simulink model "F16model"  (R2019b)
settings: Solver=ode45  StartTime=0.0  StopTime=150  RelTol=1e-7
values from neighbouring files (symbols this model uses):
  A = [ 0.005142  23.0402  -48.8785  -32.0915  0 0 0 0 0 ... (first row only)    [Final_projectMCT.m]
  B = [  1.585175  1.585175 -1.049275  -1.049275  0 0 ... (first row only)    [Final_projectMCT.m]
  KF = inv(G)*Bs'*S    [Final_projectMCT.m]
settings Model: Creator=harshireddy  LastModifiedBy=jyoth
settings SFSimCC: CustomCodeUndefinedFunction=UseInterfaceOnly

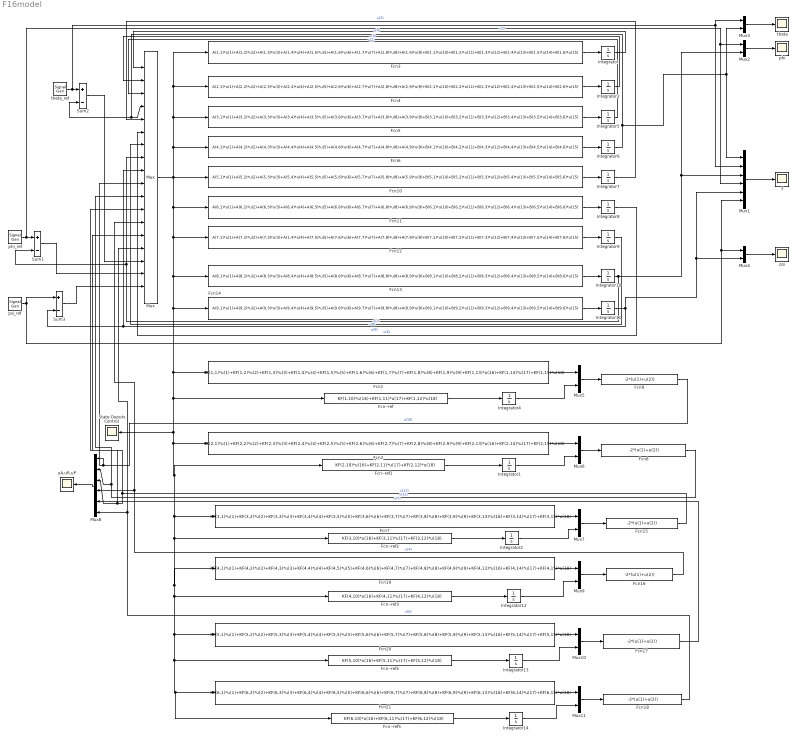
== system F16model ==
  Fcn--ref : Fcn  Expr=KF(1,10)*u(16)+KF(1,11)*u(17)+KF(1,12)*u(18)
  Fcn--ref1 : Fcn  Expr=KF(2,10)*u(16)+KF(2,11)*u(17)+KF(2,12)*u(18)
  Fcn--ref2 : Fcn  Expr=KF(3,10)*u(16)+KF(3,11)*u(17)+KF(3,12)*u(18)
  Fcn--ref3 : Fcn  Expr=KF(4,10)*u(16)+KF(4,11)*u(17)+KF(4,12)*u(18)
  Fcn--ref4 : Fcn  Expr=KF(5,10)*u(16)+KF(5,11)*u(17)+KF(5,12)*u(18)
  Fcn--ref5 : Fcn  Expr=KF(6,10)*u(16)+KF(6,11)*u(17)+KF(6,12)*u(18)
  Fcn1 : Fcn  Expr=KF(1,1)*u(1)+KF(1,2)*u(2)+KF(1,3)*u(3)+KF(1,4)*u(4)+KF(1,5)*u(5)+KF(1,6)*u(6)+KF(1,7)*u(7)+KF(1,8)*u(8)+KF(1,9)*u(9)+KF(1,13)*u(16)+KF(1,14)*u(17)+KF(1,15)*u(18)
  Fcn10 : Fcn  Expr=A(5,1)*u(1)+A(5,2)*u(2)+A(5,3)*u(3)+A(5,4)*u(4)+A(5,5)*u(5)+A(5,6)*u(6)+A(5,7)*u(7)+A(5,8)*u(8)+A(5,9)*u(9)+B(5,1)*u(10)+B(5,2)*u(11)+B(5,3)*u(12)+B(5,4)*u(13)+B(5,5)*u(14)+B(5,6)*u(15)
  Fcn11 : Fcn  Expr=A(6,1)*u(1)+A(6,2)*u(2)+A(6,3)*u(3)+A(6,4)*u(4)+A(6,5)*u(5)+A(6,6)*u(6)+A(6,7)*u(7)+A(6,8)*u(8)+A(6,9)*u(9)+B(6,1)*u(10)+B(6,2)*u(11)+B(6,3)*u(12)+B(6,4)*u(13)+B(6,5)*u(14)+B(6,6)*u(15)
  Fcn12 : Fcn  Expr=A(7,1)*u(1)+A(7,2)*u(2)+A(7,3)*u(3)+A(1,4)*u(4)+A(7,5)*u(5)+A(7,6)*u(6)+A(7,7)*u(7)+A(7,8)*u(8)+A(7,9)*u(9)+B(7,1)*u(10)+B(7,2)*u(11)+B(7,3)*u(12)+B(7,4)*u(13)+B(7,5)*u(14)+B(7,6)*u(15)
  Fcn13 : Fcn  Expr=A(8,1)*u(1)+A(8,2)*u(2)+A(8,3)*u(3)+A(8,4)*u(4)+A(8,5)*u(5)+A(8,6)*u(6)+A(8,7)*u(7)+A(8,8)*u(8)+A(8,9)*u(9)+B(8,1)*u(10)+B(8,2)*u(11)+B(8,3)*u(12)+B(8,4)*u(13)+B(8,5)*u(14)+B(8,6)*u(15)
  Fcn14 : Fcn  Expr=A(9,1)*u(1)+A(9,2)*u(2)+A(9,3)*u(3)+A(9,4)*u(4)+A(9,5)*u(5)+A(9,6)*u(6)+A(9,7)*u(7)+A(9,8)*u(8)+A(9,9)*u(9)+B(9,1)*u(10)+B(9,2)*u(11)+B(9,3)*u(12)+B(9,4)*u(13)+B(9,5)*u(14)+B(9,6)*u(15)
  Fcn{8..9,15..18} (6 alike) : Fcn  Expr=-2*(u(1)+u(2))
  Fcn19 : Fcn  Expr=KF(4,1)*u(1)+KF(4,2)*u(2)+KF(4,3)*u(3)+KF(4,4)*u(4)+KF(4,5)*u(5)+KF(4,6)*u(6)+KF(4,7)*u(7)+KF(4,8)*u(8)+KF(4,9)*u(9)+KF(4,13)*u(16)+KF(4,14)*u(17)+KF(4,15)*u(18)
  Fcn2 : Fcn  Expr=KF(2,1)*u(1)+KF(2,2)*u(2)+KF(2,3)*u(3)+KF(2,4)*u(4)+KF(2,5)*u(5)+KF(2,6)*u(6)+KF(2,7)*u(7)+KF(2,8)*u(8)+KF(2,9)*u(9)+KF(2,13)*u(16)+KF(2,14)*u(17)+KF(2,15)*u(18)
  Fcn20 : Fcn  Expr=KF(5,1)*u(1)+KF(5,2)*u(2)+KF(5,3)*u(3)+KF(5,4)*u(4)+KF(5,5)*u(5)+KF(5,6)*u(6)+KF(5,7)*u(7)+KF(5,8)*u(8)+KF(5,9)*u(9)+KF(5,13)*u(16)+KF(5,14)*u(17)+KF(5,15)*u(18)
  Fcn21 : Fcn  Expr=KF(6,1)*u(1)+KF(6,2)*u(2)+KF(6,3)*u(3)+KF(6,4)*u(4)+KF(6,5)*u(5)+KF(6,6)*u(6)+KF(6,7)*u(7)+KF(6,8)*u(8)+KF(6,9)*u(9)+KF(6,13)*u(16)+KF(6,14)*u(17)+KF(6,15)*u(18)
  Fcn3 : Fcn  Expr=A(1,1)*u(1)+A(1,2)*u(2)+A(1,3)*u(3)+A(1,4)*u(4)+A(1,5)*u(5)+A(1,6)*u(6)+A(1,7)*u(7)+A(1,8)*u(8)+A(1,9)*u(9)+B(1,1)*u(10)+B(1,2)*u(11)+B(1,3)*u(12)+B(1,4)*u(13)+B(1,5)*u(14)+B(1,6)*u(15)
  Fcn4 : Fcn  Expr=A(2,1)*u(1)+A(2,2)*u(2)+A(2,3)*u(3)+A(2,4)*u(4)+A(2,5)*u(5)+A(2,6)*u(6)+A(2,7)*u(7)+A(2,8)*u(8)+A(2,9)*u(9)+B(2,1)*u(10)+B(2,2)*u(11)+B(2,3)*u(12)+B(2,4)*u(13)+B(2,5)*u(14)+B(2,6)*u(15)
  Fcn5 : Fcn  Expr=A(3,1)*u(1)+A(3,2)*u(2)+A(3,3)*u(3)+A(3,4)*u(4)+A(3,5)*u(5)+A(3,6)*u(6)+A(3,7)*u(7)+A(3,8)*u(8)+A(3,9)*u(9)+B(3,1)*u(10)+B(3,2)*u(11)+B(3,3)*u(12)+B(3,4)*u(13)+B(3,5)*u(14)+B(3,6)*u(15)
  Fcn6 : Fcn  Expr=A(4,1)*u(1)+A(4,2)*u(2)+A(4,3)*u(3)+A(4,4)*u(4)+A(4,5)*u(5)+A(4,6)*u(6)+A(4,7)*u(7)+A(4,8)*u(8)+A(4,9)*u(9)+B(4,1)*u(10)+B(4,2)*u(11)+B(4,3)*u(12)+B(4,4)*u(13)+B(4,5)*u(14)+B(4,6)*u(15)
  Fcn7 : Fcn  Expr=KF(3,1)*u(1)+KF(3,2)*u(2)+KF(3,3)*u(3)+KF(3,4)*u(4)+KF(3,5)*u(5)+KF(3,6)*u(6)+KF(3,7)*u(7)+KF(3,8)*u(8)+KF(3,9)*u(9)+KF(3,13)*u(16)+KF(3,14)*u(17)+KF(3,15)*u(18)
  Integrator{,1..14} (15 alike) : Integrator
  Mux : Mux  Inputs=18
  Mux1 : Mux  Inputs=6
  Mux{2..7,9..11} (9 alike) : Mux  Inputs=2
  Mux8 : Mux  Inputs=6
  State Ouputs Control : Scope
  Sum1 : Sum  Inputs=+-
  Sum2 : Sum  Inputs=+-
  Sum3 : Sum  Inputs=+-
  Y : Scope
  phi : Scope
  phi_ref : SignalGenerator  WaveForm=square  Amplitude=0.1  Frequency=0.02
  psi : Scope
  psi_ref : SignalGenerator  WaveForm=square  Amplitude=0.02  Frequency=0.02
  theta : Scope
  theta_ref : SignalGenerator  WaveForm=square  Amplitude=0.1  Frequency=0.02
  uA,uR,uP : Scope
  wires:
  Fcn20/1 -> Mux10/1
  Integrator7/1 -> Mux/5  "u(5)"
  Fcn12/1 -> Integrator9/1
  Integrator6/1 -> Mux3/2, Mux1/1, Mux/4, Sum2/2  "u(4)"
  Fcn18/1 -> Mux/15, Mux8/6  "u(6)"
  Fcn13/1 -> Integrator10/1
  Integrator8/1 -> Mux/6  "u(6)"
  Fcn11/1 -> Integrator8/1
  Integrator/1 -> Mux/1  "u(1)"
  Fcn14/1 -> Integrator11/1
  Fcn9/1 -> Mux/10, Mux8/1  "u(10)"
  Fcn4/1 -> Integrator3/1
  Integrator10/1 -> Mux2/2, Mux1/3, Mux/8, Sum1/2  "u(8)"
  Integrator14/1 -> Mux11/2
  Mux2/1 -> phi/1
  Fcn8/1 -> Mux/11, Mux8/2  "u(11)"
  theta_ref/1 -> Mux1/2, Mux3/1, Sum2/1
  Fcn5/1 -> Integrator5/1
  Sum2/1 -> Mux/16
  Sum3/1 -> Mux/18
  Fcn2/1 -> Mux6/1
  psi_ref/1 -> Mux1/6, Mux4/1, Sum3/1
  Fcn10/1 -> Integrator7/1
  Fcn--ref4/1 -> Integrator13/1
  Integrator3/1 -> Mux/2  "u(2)"
  Mux7/1 -> Fcn15/1
  phi_ref/1 -> Mux2/1, Mux1/4, Sum1/1
  Mux6/1 -> Fcn8/1
  Fcn--ref1/1 -> Integrator1/1
  Fcn--ref2/1 -> Integrator2/1
  Mux9/1 -> Fcn16/1
  Mux5/1 -> Fcn9/1
  Mux11/1 -> Fcn18/1
  Fcn--ref/1 -> Integrator4/1
  Fcn15/1 -> Mux/14, Mux8/3, Mux/12  "u(12)"
  Sum1/1 -> Mux/17
  Fcn3/1 -> Integrator/1
  Fcn6/1 -> Integrator6/1
  Integrator11/1 -> Mux/9, Sum3/2, Mux1/5, Mux4/2  "u(9)"
  Mux8/1 -> uA,uR,uP/1
  Mux/1 -> Fcn11/1, Fcn12/1, Fcn13/1, State Ouputs Control/1, Fcn--ref5/1, Fcn21/1, Fcn--ref4/1, Fcn20/1, Fcn--ref3/1, Fcn19/1, Fcn--ref2/1, Fcn7/1, Fcn--ref1/1, Fcn2/1, Fcn--ref/1, Fcn1/1, Fcn14/1, Fcn10/1, Fcn6/1, Fcn5/1, Fcn4/1, Fcn3/1
  Fcn21/1 -> Mux11/1
  Integrator5/1 -> Mux/3  "u(3)"
  Mux1/1 -> Y/1
  Integrator13/1 -> Mux10/2
  Integrator9/1 -> Mux/7  "u(7)"
  Mux4/1 -> psi/1
  Fcn--ref5/1 -> Integrator14/1
  Integrator12/1 -> Mux9/2
  Fcn19/1 -> Mux9/1
  Integrator4/1 -> Mux5/2
  Fcn16/1 -> Mux/13, Mux8/4  "u(4)"
  Fcn17/1 -> Mux8/5  "u(5)"
  Integrator1/1 -> Mux6/2
  Integrator2/1 -> Mux7/2
  Fcn1/1 -> Mux5/1
  Mux10/1 -> Fcn17/1
  Fcn7/1 -> Mux7/1
  Fcn--ref3/1 -> Integrator12/1
  Mux3/1 -> theta/1
